simulink model "First"  (R2015b)
settings: Solver=FixedStepAuto  StartTime=0.0  StopTime=inf  FixedStep=0.0000001  RelTol=1e-3
settings Model: Creator=User  LastModifiedBy=User

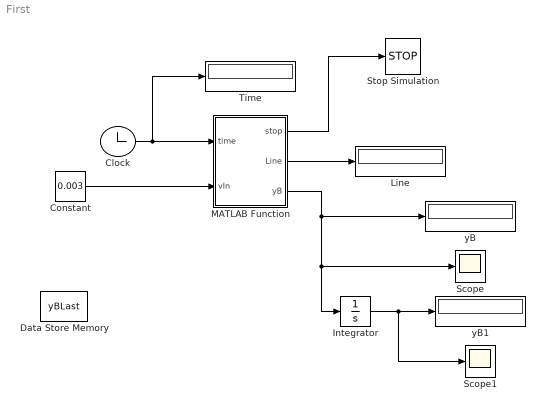
== system First ==
  Clock : Clock
  Constant : Constant  Value=0.003
  Data Store Memory : DataStoreMemory  DataStoreName=yBLast  ReadBeforeWriteMsg=warning  WriteAfterWriteMsg=warning  WriteAfterReadMsg=warning  OutDataTypeStr=double
  Integrator : Integrator
  Line : Display
  MATLAB Function : MATLAB Function  TreatAsAtomicUnit=on
  Scope : Scope
  Scope1 : Scope
  Stop Simulation : Stop
  Time : Display
  yB : Display
  yB1 : Display
  wires:
  Clock/1 -> Time/1, MATLAB Function/1(time)
  Constant/1 -> MATLAB Function/2(vIn)
  MATLAB Function/1(stop) -> Stop Simulation/1
  MATLAB Function/2(Line) -> Line/1
  MATLAB Function/3(yB) -> Integrator/1, Scope/1, yB/1
  Integrator/1 -> Scope1/1, yB1/1

== matlab function First/MATLAB Function ==
  data: time input; stop output; vIn input; Line output; yB output; yBLast data_store_memory
function [stop,Line,yB] = fcn(time,vIn)
%#codegen

global yBLast;
%persistent yBL;
Line = vIn*time;
if (Line >= 0.1)
    stop = 1;
else
    stop = 0;
end

m = 0.000221;
pi = 3.1415926535;
alfaG = 45;
gammaG = 90-alfaG;
gammaR = (gammaG*pi)/180;
E = 2*(10^11);
d = 0.001;
dIn = 0.0008;
s = pi*(d/2)*(d/2)*Line;
rho = 1300;

%needleF =  0.5; 
cF  = 1.15;%0.82;%(2*(needleF))/(rho*vIn*vIn*s);

envF   = cF*s*( (rho*vIn*vIn)/2  );  
envFp  = envF*cos(gammaR);
iIx    = ((Line)*((d^3) - (dIn^3)))/12;
if iIx == 0
    yB = 0;
else
yB     =   1000*(envFp*((Line)^3))/(3*E*iIx);
yBLast = yB;
end
end
